simulink model "gcu_flat"  (R2025b)
settings: Solver=FixedStepAuto  StartTime=0.0  StopTime=10.0  RelTol=1e-3
model workspace (MAT data in the model file):
  drone_idx = 1
undefined symbols (not defined in the file): fctrl, quadcop, traj, Ts_gcs
settings Model: DataDictionary=project.sldd  ParameterArgumentNames=drone_idx  Creator=Nick  LastModifiedBy=Rakete

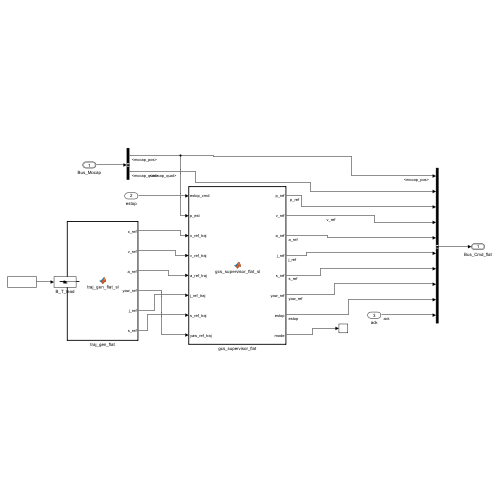
[thumbnail: Simulink's stored preview of the top-level diagram]
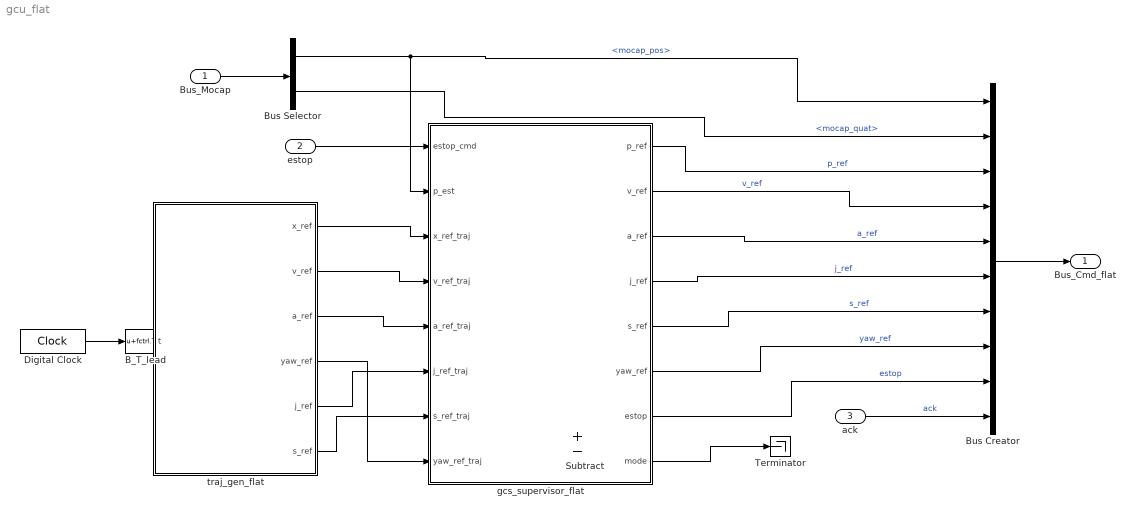
== system gcu_flat ==
  Bus_Mocap : Inport  OutDataTypeStr=Bus: Bus_Mocap
  estop : Inport  Port=2  OutDataTypeStr=uint8
  ack : Inport  Port=3  OutDataTypeStr=boolean  PortDimensions=1
  B_T_lead : Bias  Bias=fctrl.T_lead  SaturateOnIntegerOverflow=off
  Bus Creator : BusCreator  Inputs=10  OutDataTypeStr=Bus: Bus_Cmd_flat
      settings: InheritFromInputs=off
  Bus Selector : BusSelector  OutputSignals=mocap_pos,mocap_quat
  Digital Clock : DigitalClock  SampleTime=Ts_gcs
  Subtract : Sum  Inputs=+-
  Terminator : Terminator
  gcs_supervisor_flat : MATLAB Function  TreatAsAtomicUnit=on  SystemSampleTime=Ts_gcs
  traj_gen_flat : MATLAB Function  TreatAsAtomicUnit=on
  Bus_Cmd_flat : Outport  OutDataTypeStr=Bus: Bus_Cmd_flat
  wires:
  traj_gen_flat/1(x_ref) -> gcs_supervisor_flat/3(x_ref_traj)
  Bus_Mocap/1 -> Bus Selector/1
  traj_gen_flat/3(a_ref) -> gcs_supervisor_flat/5(a_ref_traj)
  estop/1 -> gcs_supervisor_flat/1(estop_cmd)
  Bus Selector/2 -> Bus Creator/2  "<mocap_quat>"
  traj_gen_flat/2(v_ref) -> gcs_supervisor_flat/4(v_ref_traj)
  Bus Selector/1 -> gcs_supervisor_flat/2(p_est), Bus Creator/1  "<mocap_pos>"
  traj_gen_flat/4(yaw_ref) -> gcs_supervisor_flat/8(yaw_ref_traj)
  traj_gen_flat/5(j_ref) -> gcs_supervisor_flat/6(j_ref_traj)
  traj_gen_flat/6(s_ref) -> gcs_supervisor_flat/7(s_ref_traj)
  gcs_supervisor_flat/1(p_ref) -> Bus Creator/3  "p_ref"
  gcs_supervisor_flat/2(v_ref) -> Bus Creator/4  "v_ref"
  gcs_supervisor_flat/3(a_ref) -> Bus Creator/5  "a_ref"
  gcs_supervisor_flat/4(j_ref) -> Bus Creator/6  "j_ref"
  gcs_supervisor_flat/5(s_ref) -> Bus Creator/7  "s_ref"
  gcs_supervisor_flat/6(yaw_ref) -> Bus Creator/8  "yaw_ref"
  gcs_supervisor_flat/7(estop) -> Bus Creator/9  "estop"
  ack/1 -> Bus Creator/10  "ack"
  gcs_supervisor_flat/8(mode) -> Terminator/1
  Bus Creator/1 -> Bus_Cmd_flat/1
  Digital Clock/1 -> B_T_lead/1
  B_T_lead/1 -> traj_gen_flat/1(t)

== matlab function gcu_flat/traj_gen_flat ==
  data: t input; x_ref output; v_ref output; a_ref output; yaw_ref output; j_ref output; s_ref output; traj parameter; quadcop parameter; drone_idx parameter
function [x_ref, v_ref, a_ref, yaw_ref, j_ref, s_ref] = traj_gen_flat_sl(t, traj, quadcop, drone_idx)
%#codegen
% WRAPPER -- code liegt in
% scripts\functions\traj_gen.m - dieser Block ruft sie nur auf.
% drone_idx: Modellargument von gcu_flat (Scheibe der Drohne im geteilten traj,
% siehe bench_init_fcn) -- Einzeldrohne: drone_idx = 1.
% Folgeregler als asymptotisches Model Matching mit dem Referenzmodell (p_r, v_r, a_r):
% Ruck und Snap werden fuer Tabellen UND Wegpunkte nicht vorgesteuert.
[x_ref, v_ref, a_ref, yaw_ref] = traj_gen(t, traj, quadcop, drone_idx);
j_ref = zeros(3, 1);
s_ref = zeros(3, 1);
end

== matlab function gcu_flat/gcs_supervisor_flat ==
  data: estop_cmd input; p_ref output; p_est input; x_ref_traj input; v_ref_traj input; a_ref_traj input; j_ref_traj input; s_ref_traj input; yaw_ref_traj input; v_ref output; a_ref output; j_ref output; s_ref output; yaw_ref output; estop output; mode output; supervisor parameter
function [p_ref, v_ref, a_ref, j_ref, s_ref, yaw_ref, estop, mode] = gcs_supervisor_flat_sl(estop_cmd, p_est, x_ref_traj, v_ref_traj, a_ref_traj, j_ref_traj, s_ref_traj, yaw_ref_traj, supervisor)
%#codegen
% WRAPPER — code liegt in
% scripts\flatness\gcs_supervisor_flat.m - dieser Block ruft sie nur auf
[p_ref, v_ref, a_ref, j_ref, s_ref, yaw_ref, estop, mode] = gcs_supervisor_flat(estop_cmd, p_est, x_ref_traj, v_ref_traj, a_ref_traj, j_ref_traj, s_ref_traj, yaw_ref_traj, supervisor);
end
